simulink model "CCS_3"  (R2019b)
settings: Solver=VariableStepAuto  StartTime=0.0  StopTime=0.25  RelTol=1e-3
libraries: simulink x1
settings Model: Creator=Administrator  LastModifiedBy=Administrator

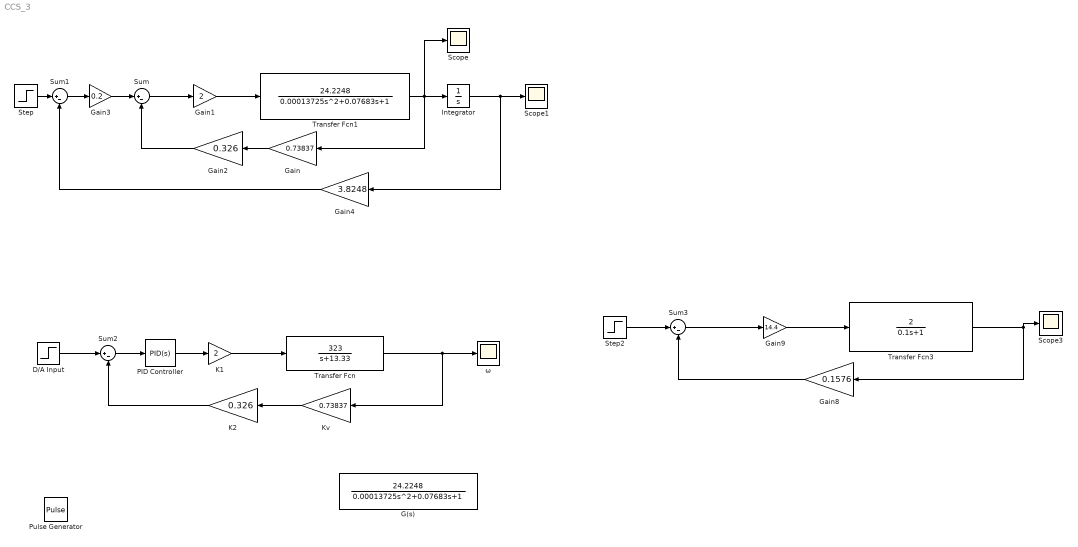
== system CCS_3 ==
  D/A Input : Step  Time=0  SampleTime=0
  G(s) : TransferFcn  Numerator=[24.2248]  Denominator=[0.00013725 0.07683 1]
  Gain : Gain  Gain=0.73837
  Gain1 : Gain  Gain=2
  Gain2 : Gain  Gain=0.326
  Gain3 : Gain  Gain=0.2
  Gain4 : Gain  Gain=3.8248
  Gain8 : Gain  Gain=0.1576
  Gain9 : Gain  Gain=14.4
  Integrator : Integrator
  K1 : Gain  Gain=2
  K2 : Gain  Gain=0.326
  Kv : Gain  Gain=0.73837
  PID Controller : simulink/Continuous/PID Controller  Controller=PID  Form=Parallel  TimeDomain=Continuous-time  SampleTime=-1  IntegratorMethod=Forward Euler  FilterMethod=Forward Euler  ControllerParametersSource=internal  P=1  I=0  D=0  UseFilter=on  N=100  TunerSelectOption=Transfer Function Based (PID Tuner App)  InitialConditionSource=internal  InitialConditionForIntegrator=0  InitialConditionForFilter=0  DifferentiatorICPrevScaledInput=0  ExternalReset=none  TrackingMode=off  Kt=1  LimitOutput=off  UpperSaturationLimit=inf  LowerSaturationLimit=-inf  LinearizeAsGain=on  AntiWindupMode=none  Kb=1  POutMin=[]  POutMax=[]  IOutMin=[]  IOutMax=[]  DOutMin=[]  DOutMax=[]  NOutMin=[]  NOutMax=[]  SumOutMin=[]  SumOutMax=[]  SaturationOutMin=[]  SaturationOutMax=[]  PParamMin=[]  PParamMax=[]  IParamMin=[]  IParamMax=[]  DParamMin=[]  DParamMax=[]  NParamMin=[]  NParamMax=[]  KbParamMin=[]  KbParamMax=[]  KtParamMin=[]  KtParamMax=[]  KbOutMin=[]  KbOutMax=[]  KtOutMin=[]  KtOutMax=[]  IntegratorOutMin=[]  IntegratorOutMax=[]  FilterOutMin=[]  FilterOutMax=[]  SumI1OutMin=[]  SumI1OutMax=[]  SumI2OutMin=[]  SumI2OutMax=[]  SumI3OutMin=[]  SumI3OutMax=[]  SumI4OutMin=[]  SumI4OutMax=[]  SumDOutMin=[]  SumDOutMax=[]  DifferentiatorOutMin=[]  DifferentiatorOutMax=[]  FilterDiffOutCoefMin=[]  FilterDiffOutCoefMax=[]  ReciprocalOutMin=[]  ReciprocalOutMax=[]  SumDenOutMin=[]  SumDenOutMax=[]  SumNumOutMin=[]  SumNumOutMax=[]  DivideOutMin=[]  DivideOutMax=[]  IntegratorContinuousStateAttributes=''  IntegratorStateMustResolveToSignalObject=off  IntegratorRTWStateStorageClass=Auto  FilterContinuousStateAttributes=''  FilterStateMustResolveToSignalObject=off  FilterRTWStateStorageClass=Auto  ParallelPVariant=InternalParameters  IdealPVariant=Disabled  IVariant=InternalParameters  DVariant=InternalParameters  IntegratorVariant=Continuous  SatVariant=Disabled  AWVariant=Passthrough  PCopyVariant=Disabled  TRVariant=Disabled  FdbkBlocksVariant=Forward  IdealPFdbkVariant=Disabled  SatFdbkVariant=Disabled  DerivativeFilterVariant=ContFilter  NVariant=InternalParameters  NCopyVariant=Disabled  FilterICVariant=InternalICsFilter  IntegratorICVariant=InternalICs  ExternalResetVariant=Disabled  TRSumVariant=Passthrough  SumFdbkVariant=Disabled  SumVariant=Sum_PID
  Pulse Generator : DiscretePulseGenerator  PulseType=Time based  Period=10  PulseWidth=5
  Scope : Scope
  Scope1 : Scope
  Scope3 : Scope
  Step : Step  Time=0  After=5  SampleTime=0
  Step2 : Step  Time=0  After=4  SampleTime=0
  Sum{,1..3} (4 alike) : Sum  Inputs=|+-
  Transfer Fcn : TransferFcn  Numerator=[323]  Denominator=[1 13.33]
  Transfer Fcn1 : TransferFcn  Numerator=[24.2248]  Denominator=[0.00013725 0.07683 1]
  Transfer Fcn3 : TransferFcn  Numerator=[2]  Denominator=[0.1 1]
  ω : Scope
  wires:
  Gain/1 -> Gain2/1
  Gain2/1 -> Sum/2
  Gain1/1 -> Transfer Fcn1/1
  Transfer Fcn1/1 -> Integrator/1, Gain/1, Scope/1
  Sum/1 -> Gain1/1
  Integrator/1 -> Gain4/1, Scope1/1
  Gain3/1 -> Sum/1
  Step/1 -> Sum1/1
  Sum1/1 -> Gain3/1
  Gain4/1 -> Sum1/2
  Kv/1 -> K2/1
  K2/1 -> Sum2/2
  Sum2/1 -> PID Controller/1
  PID Controller/1 -> K1/1
  Step2/1 -> Sum3/1
  Gain9/1 -> Transfer Fcn3/1
  Transfer Fcn3/1 -> Scope3/1, Gain8/1
  Gain8/1 -> Sum3/2
  Sum3/1 -> Gain9/1
  K1/1 -> Transfer Fcn/1
  Transfer Fcn/1 -> ω/1, Kv/1
  D/A Input/1 -> Sum2/1
